simulink model "RLCmodel"  (Simulink 8.8)
settings: Solver=ode3  StartTime=0.0  StopTime=0.01  FixedStep=0.00001  RelTol=1e-3  EnableMultiTasking=on
InitFcn:
  | initRLC
values from neighbouring files (symbols this model uses):
  A = [-R/L -1/L;1/Cap 0]    [initRLC.m]
  Ad = eye(2)+A*dT    [initRLC.m]
  B = [1/L 0]'    [initRLC.m]
  Bd = B*dT    [initRLC.m]
  C = [1 0]    [initRLC.m]
  Cap = 1e-6    (= 1e-06)    [initRLC.m]
  Cd = C    [initRLC.m]
  D = 0    [initRLC.m]
  Dd = D    (= 0)    [initRLC.m]
  dT = 0.00001    (= 1e-05)    [initRLC.m]
  L = 10e-3    (= 0.01)    [initRLC.m]
  R = 50    [initRLC.m]
settings Model: Creator=ageorgip  LastModifiedBy=igeorgie
settings OptimizationCC: ExpressionDepthLimit=2147483647  InitFltsAndDblsToZero=on
settings DebuggingCC: SolverPrmCheckMsg=warning
settings GRTTargetCC: GeneratePreprocessorConditionals=Use local settings

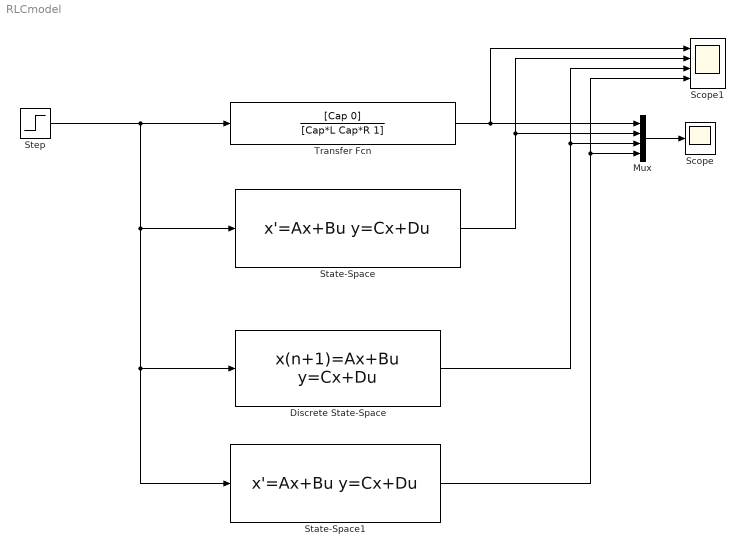
== system RLCmodel ==
  Discrete State-Space : DiscreteStateSpace  A=Ad  B=Bd  C=Cd  D=Dd  SampleTime=dT
  Mux : Mux
  Scope : Scope
  Scope1 : Scope  NumInputPorts=4
  State-Space : StateSpace  A=A  B=B  C=C  D=D  X0=0
  State-Space1 : StateSpace  A=[0 1;-1/(L*Cap) -R/L]  B=[0 1]'  C=[0 1/L]  D=0  X0=0
  Step : Step  Time=0.0001
  Transfer Fcn : TransferFcn  Numerator=[Cap 0]  Denominator=[Cap*L Cap*R 1]
  wires:
  Transfer Fcn/1 -> Mux/1, Scope1/1
  State-Space/1 -> Mux/2, Scope1/2
  Discrete State-Space/1 -> Mux/3, Scope1/3
  Mux/1 -> Scope/1
  State-Space1/1 -> Mux/4, Scope1/4
  Step/1 -> Transfer Fcn/1, State-Space/1, Discrete State-Space/1, State-Space1/1
